simulink model "q10"  (R2016a)
settings: Solver=VariableStepAuto  StartTime=0.0  StopTime=100  RelTol=1e-3
libraries: simulink x1
settings Model: Creator=derakhshani4476  LastModifiedBy=derakhshani4476

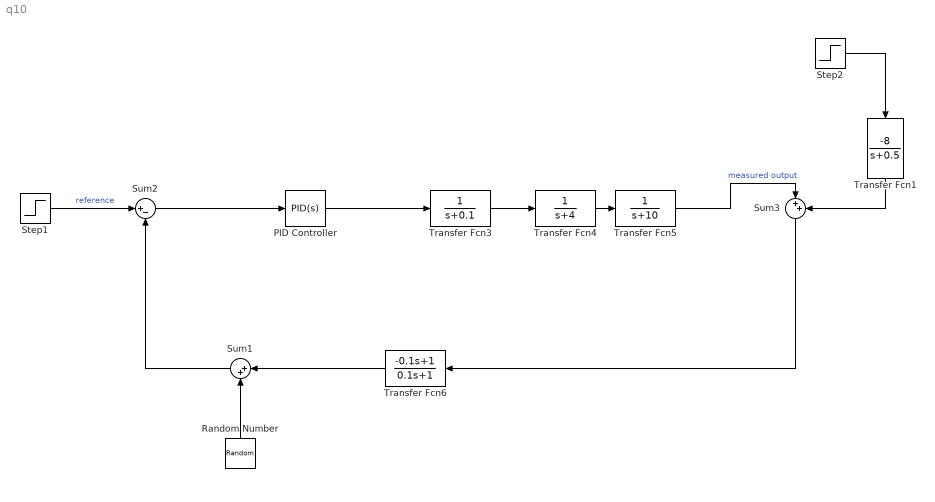
== system q10 ==
  PID Controller : simulink/Continuous/PID Controller  Controller=PID  TimeDomain=Continuous-time  SampleTime=-1  IntegratorMethod=Forward Euler  FilterMethod=Forward Euler  Form=Parallel  UseFilter=on  ControllerParametersSource=internal  P=59.04  I=20.41  D=15.64  N=100  InitialConditionSource=internal  InitialConditionForIntegrator=0  InitialConditionForFilter=0  ExternalReset=none  LimitOutput=off  UpperSaturationLimit=inf  LowerSaturationLimit=-inf  LinearizeAsGain=on  AntiWindupMode=none  Kb=1  TrackingMode=off  Kt=1  PParamMin=[]  PParamMax=[]  IParamMin=[]  IParamMax=[]  DParamMin=[]  DParamMax=[]  NParamMin=[]  NParamMax=[]  KbParamMin=[]  KbParamMax=[]  KtParamMin=[]  KtParamMax=[]  POutMin=[]  POutMax=[]  IOutMin=[]  IOutMax=[]  DOutMin=[]  DOutMax=[]  NOutMin=[]  NOutMax=[]  KbOutMin=[]  KbOutMax=[]  KtOutMin=[]  KtOutMax=[]  IntegratorOutMin=[]  IntegratorOutMax=[]  FilterOutMin=[]  FilterOutMax=[]  SumOutMin=[]  SumOutMax=[]  SumI1OutMin=[]  SumI1OutMax=[]  SumI2OutMin=[]  SumI2OutMax=[]  SumI3OutMin=[]  SumI3OutMax=[]  SumDOutMin=[]  SumDOutMax=[]  SaturationOutMin=[]  SaturationOutMax=[]  IntegratorContinuousStateAttributes=''  IntegratorStateMustResolveToSignalObject=off  IntegratorRTWStateStorageClass=Auto  FilterContinuousStateAttributes=''  FilterStateMustResolveToSignalObject=off  FilterRTWStateStorageClass=Auto  DifferentiatorICPrevScaledInput=0  DifferentiatorOutMin=[]  DifferentiatorOutMax=[]
  Random Number : RandomNumber  Variance=36  SampleTime=0.1
  Step1 : Step  Time=0  After=100  SampleTime=0
  Step2 : Step  Before=1  After=10  SampleTime=0
  Sum1 : Sum  Inputs=|++
  Sum2 : Sum  Inputs=|+-
  Sum3 : Sum  Inputs=|++
  Transfer Fcn1 : TransferFcn  Numerator=[-8]  Denominator="[ 1 0.5  ]"
  Transfer Fcn3 : TransferFcn  Denominator="[ 1 0.1  ]"
  Transfer Fcn4 : TransferFcn  Denominator="[ 1 4  ]"
  Transfer Fcn5 : TransferFcn  Denominator="[ 1 10  ]"
  Transfer Fcn6 : TransferFcn  Numerator=[-0.1 1]  Denominator=[0.1 1]
  wires:
  Step1/1 -> Sum2/1  "reference"
  Transfer Fcn3/1 -> Transfer Fcn4/1
  Transfer Fcn4/1 -> Transfer Fcn5/1
  Random Number/1 -> Sum1/2
  Transfer Fcn6/1 -> Sum1/1
  Sum1/1 -> Sum2/2
  Transfer Fcn5/1 -> Sum3/1  "measured output"
  Transfer Fcn1/1 -> Sum3/2
  Step2/1 -> Transfer Fcn1/1
  Sum3/1 -> Transfer Fcn6/1
  PID Controller/1 -> Transfer Fcn3/1
  Sum2/1 -> PID Controller/1
